simulink model "Trajectory_Tracking_Control_Structure3_Modifying"  (R2017b)
settings: Solver=VariableStepAuto  StartTime=0  StopTime=times(end)  RelTol=1e-6
values from neighbouring files (symbols this model uses):
  a_piecewise = zeros(max(DOF_a_piecewise),length(DOF_a_piecewise))    [Trajectory_Generator_Minimum_Snap.m]
  b_piecewise = zeros(max(DOF_b_piecewise),length(DOF_b_piecewise))    [Trajectory_Generator_Minimum_Snap.m]
  c_piecewise = zeros(max(DOF_c_piecewise),length(DOF_c_piecewise))    [Trajectory_Generator_Minimum_Snap.m]
  d_piecewise = zeros(max(DOF_d_piecewise),length(DOF_d_piecewise))    [Trajectory_Generator_Minimum_Snap.m]
settings Model: Creator=chenjiasheng  LastModifiedBy=chenjiasheng

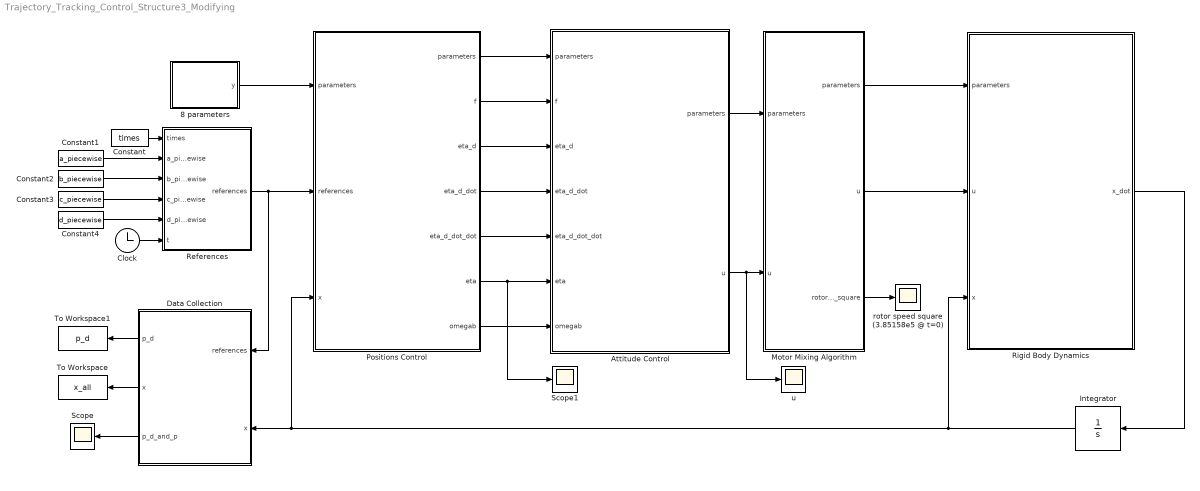
== system Trajectory_Tracking_Control_Structure3_Modifying ==
  8 parameters : MATLAB Function  TreatAsAtomicUnit=on
  Attitude Control : MATLAB Function  TreatAsAtomicUnit=on
  Clock : Clock
  Constant : Constant  Value=times
  Constant1 : Constant  Value=a_piecewise
  Constant2 : Constant  Value=b_piecewise
  Constant3 : Constant  Value=c_piecewise
  Constant4 : Constant  Value=d_piecewise
  Data Collection : MATLAB Function  TreatAsAtomicUnit=on
  Integrator : Integrator  InitialCondition=[0 0 0, 0 0 0, 0 0 0, 0 0 0]  ContinuousStateAttributes='x'
  Motor Mixing Algorithm : MATLAB Function  TreatAsAtomicUnit=on
  Positions Control : MATLAB Function  TreatAsAtomicUnit=on
  References : MATLAB Function  TreatAsAtomicUnit=on
  Rigid Body Dynamics : MATLAB Function  TreatAsAtomicUnit=on
  Scope : Scope
  Scope1 : Scope
  To Workspace : ToWorkspace  VariableName=x_all  SampleTime=0.01
  To Workspace1 : ToWorkspace  VariableName=p_d  SampleTime=0.01
  rotor speed square (3.85158e5 @ t=0) : Scope
  u : Scope
  wires:
  8 parameters/1(y) -> Positions Control/1("parameters ")
  References/1(references) -> Positions Control/2(references), Data Collection/1(references)
  Positions Control/1(parameters) -> Attitude Control/1("parameters ")
  Positions Control/2(f) -> Attitude Control/2(f)
  Positions Control/3(eta_d) -> Attitude Control/3(eta_d)
  Positions Control/4(eta_d_dot) -> Attitude Control/4(eta_d_dot)
  Rigid Body Dynamics/1(x_dot) -> Integrator/1
  Integrator/1 -> Rigid Body Dynamics/3(x), Positions Control/3(x), Data Collection/2("x ")
  Attitude Control/1(parameters) -> Motor Mixing Algorithm/1("parameters ")
  Attitude Control/2(u) -> u/1, Motor Mixing Algorithm/2("u ")
  Clock/1 -> References/6(t)
  Motor Mixing Algorithm/1(parameters) -> Rigid Body Dynamics/1(parameters)
  Motor Mixing Algorithm/2(u) -> Rigid Body Dynamics/2(u)
  Motor Mixing Algorithm/3(rotor_speed_square) -> rotor speed square (3.85158e5 @ t=0)/1
  Positions Control/5(eta_d_dot_dot) -> Attitude Control/5(eta_d_dot_dot)
  Positions Control/6(eta) -> Scope1/1, Attitude Control/6(eta)
  Positions Control/7(omegab) -> Attitude Control/7(omegab)
  Constant/1 -> References/1(times)
  Constant1/1 -> References/2(a_piecewise)
  Constant2/1 -> References/3(b_piecewise)
  Constant3/1 -> References/4(c_piecewise)
  Constant4/1 -> References/5(d_piecewise)
  Data Collection/1(p_d) -> To Workspace1/1
  Data Collection/3(p_d_and_p) -> Scope/1
  Data Collection/2(x) -> To Workspace/1

== matlab function Trajectory_Tracking_Control_Structure3_Modifying/Positions Control ==
  data: parameters input size=8; parameters output size=8; references input size=18; x input size=12; f output size=1; eta_d output size=3; eta_d_dot output size=3; eta_d_dot_dot output size=3; eta output size=3; omegab output size=3
 function [parameters,f,eta_d,eta_d_dot,eta_d_dot_dot,eta,omegab] =fcn(parameters,references,x)
%% kp,kd for the positions controller
Kp=diag([0 0 0]); % Kp=diag([kpx kpy kpz]) [20 30 20]
Kd=diag([0 0 0]);    % Kd=diag([kdx kdy kdz])[6 15 6]
%% allocate inputs
m=parameters(1);
g=parameters(2);
p_d=references(1:3);   % reference's positions
v_d=references(4:6);   % reference's velocities
a_d=references(7:9);   % reference's accelerations
a_d_dot=references(10:12);    % reference's jerk
a_d_dot_dot=references(13:15);% reference's snap
psi_d=references(16);         % reference's yaw angle 
psi_d_dot=references(17);     % reference's change rate of the yaw angle
psi_d_dot_dot=references(18); % reference's change rate of change rate of the yaw angle
p=x(1:3) ;     % positions 
v=x(4:6) ;     % velocities
eta=x(7:9);    % euler angle
omegab=x(10:12); 
phi=eta(1);
theta=eta(2);
psi=eta(3);
Rbn=[cos(theta)*cos(psi) sin(phi)*sin(theta)*cos(psi)-cos(phi)*sin(psi) cos(phi)*sin(theta)*cos(psi)+sin(phi)*sin(psi);
     cos(theta)*sin(psi) sin(phi)*sin(theta)*sin(psi)+cos(phi)*cos(psi) cos(phi)*sin(theta)*sin(psi)-sin(phi)*cos(psi);
     -sin(theta)         sin(phi)*cos(theta)                            cos(phi)*cos(theta)                           ];
zb=Rbn(:,3);
%% acceleration, jerk, snap control
a_c=Kp*(p_d-p)+Kd*(v_d-v)+a_d;  % acceleration of control
f=m*sqrt(a_c(1)^2+a_c(2)^2+(g+a_c(3))^2);
a=1/m*Rbn*[0 0 f]'-[0 0 g]';
a_c_dot=Kp*(v_d-v)+Kd*(a_d-a)+a_d_dot ;   % acceleration of control dot
a_dot=m/f*[a_c(1),a_c(2),a_c(3)+g]*a_c_dot*zb+f/m*cross((Rbn*omegab),zb);
a_c_dot_dot=Kp*(a_d-a)+Kd*(a_d_dot-a_dot)+a_d_dot_dot; % acceleration of control dot dot
%% define some variables to make our life easier
A=a_c(1)*sin(psi_d)-a_c(2)*cos(psi_d); 
C=a_c(1)*cos(psi_d)+a_c(2)*sin(psi_d);
D=g+a_c(3);
B=sqrt(C^2+D^2);
A_dot=sin(psi_d)*a_c_dot(1)-cos(psi_d)*a_c_dot(2)+C*psi_d_dot;                                   
C_dot=cos(psi_d)*a_c_dot(1)+sin(psi_d)*a_c_dot(2)-A*psi_d_dot;                                  
D_dot=a_c_dot(3);                                                                                
B_dot=(C*C_dot+D*D_dot)/B;  
fbmsd=2*a_c(1)*a_c_dot(1)+2*a_c(2)*a_c_dot(2)+2*(g+a_c(3))*a_c_dot(3);   % f by m square dot
%% phi_d, theta_d 
phi_d=asin(A*m/f) ;
theta_d=sign(C)*acos(D/B);
%% phi_d_dot,theta_d_dot
phi_d_dot=(sin(psi_d)*(f/m)^2-A*a_c(1))/((f/m)^2*B)*a_c_dot(1) + (-cos(psi_d)*(f/m)^2-A*a_c(2))/((f/m)^2*B)*a_c_dot(2) + (-A*D)/((f/m)^2*B)*a_c_dot(3) + C/B*psi_d_dot ;
theta_d_dot=(cos(psi_d)*D*a_c_dot(1)+sin(psi_d)*D*a_c_dot(2)-C*a_c_dot(3)-A*D*psi_d_dot)/B^2   ; 
%% phi_d_dot_dot, theta_d_dot_dot
monster11=(cos(psi_d)*psi_d_dot*(f/m)^2+sin(psi_d)*fbmsd-(A_dot*a_c(1)+A*a_c_dot(1)))*a_c_dot(1)+(sin(psi_d)*(f/m)^2-A*a_c(1))*a_c_dot_dot(1);
monster12=(-sin(psi_d)*psi_d_dot*(f/m)^2+cos(psi_d)*fbmsd+A_dot*a_c(2)+A*a_c_dot(2))*a_c_dot(2)+(cos(psi_d)*(f/m)^2+A*a_c(2))*a_c_dot_dot(2);
monster13=(A_dot*D+A*D_dot)*a_c_dot(3)+A*D*a_c_dot_dot(3);
monster1=monster11-monster12-monster13;
phi_d_dot_dot=(monster1-(B*phi_d_dot-C*psi_d_dot)*fbmsd)/((f/m)^2*B) + (C_dot*psi_d_dot+C*psi_d_dot_dot-B_dot*phi_d_dot)/B;
monster21=(-sin(psi_d)*psi_d_dot*D+cos(psi_d)*D_dot)*a_c_dot(1)+cos(psi_d)*D*a_c_dot_dot(1);
monster22=(cos(psi_d)*psi_d_dot*D+sin(psi_d)*D_dot)*a_c_dot(2)+sin(psi_d)*D*a_c_dot_dot(2);
monster23= C_dot*a_c_dot(3)+C*a_c_dot_dot(3);
monster24=(A_dot*D+A*D_dot)*psi_d_dot+A*D*psi_d_dot_dot;
monster2= monster21+monster22-monster23-monster24;
theta_d_dot_dot=monster2/B^2-2*theta_d_dot*B_dot/B;
%% output eta_d, eta_d_dot, eta_d_dot_dot                        
 % output 1-8: eight parameters  (given above)
 % output 9: f (given above)
eta_d=[phi_d;theta_d;psi_d]   ;                 % output 10-12
eta_d_dot=[phi_d_dot;theta_d_dot;psi_d_dot] ;       % output 13-15 
eta_d_dot_dot=[phi_d_dot_dot;theta_d_dot_dot;psi_d_dot_dot];% output 16-18
 % output 19-21: eta (given above)
 % output 22-24: omegab (given above)

== matlab function Trajectory_Tracking_Control_Structure3_Modifying/8 parameters ==
  data: y output size=8
function y=fcn
%% specify parameters
m=0.468;
g=9.81;
Ix=4.856*10^(-3);
Iy=4.856*10^(-3);
Iz=8.801*10^(-3);
l=0.225;
k=2.980*10^-6;
c=1.140*10^-7;
%% output
y=[m;g;Ix;Iy;Iz;l;k;c]; % output # 1-8
    
end

== matlab function Trajectory_Tracking_Control_Structure3_Modifying/Attitude Control ==
  data: parameters input size=8; parameters output size=8; f input size=1; eta_d input size=3; eta_d_dot input size=3; eta_d_dot_dot input size=3; eta input size=3; omegab input size=3; u output size=4
function [parameters,u]=fcn(parameters,f,eta_d,eta_d_dot,eta_d_dot_dot,eta,omegab)
%% kp, kd for the attitude control
KP=diag([150 150 150]); % kp_phi, kp_theta, kp_psi
KD=diag([22 22 22]); % kd_phi, kd_theta, kd_psi
%% allocate inputs
M=diag([parameters(3), parameters(4), parameters(5)]);
phi=eta(1);
theta=eta(2);
psi=eta(3);
eta_dot=[1 sin(phi)*tan(theta) cos(phi)*tan(theta);
         0 cos(phi)            -sin(phi);
         0 sin(phi)/cos(theta) cos(phi)/cos(theta)]*omegab;
phi_dot=eta_dot(1);
theta_dot=eta_dot(2);
psi_dot=eta_dot(3);
%% get taub
eta_c_dot_dot=KP*(eta_d-eta)+KD*(eta_d_dot-eta_dot)+eta_d_dot_dot;
phi_c_dot_dot=eta_c_dot_dot(1);
theta_c_dot_dot=eta_c_dot_dot(2);
psi_c_dot_dot=eta_c_dot_dot(3);
p_c_dot=phi_c_dot_dot-psi_c_dot_dot*sin(theta)-theta_dot*psi_dot*cos(theta);
q_c_dot=theta_c_dot_dot*cos(phi)+psi_c_dot_dot*sin(phi)*cos(theta)-phi_dot*theta_dot*sin(phi)+phi_dot*psi_dot*cos(phi)*cos(theta)-theta_dot*psi_dot*sin(phi)*sin(theta);
r_c_dot=-theta_c_dot_dot*sin(phi)+psi_c_dot_dot*cos(phi)*cos(theta)-phi_dot*theta_dot*cos(phi)-phi_dot*psi_dot*sin(phi)*cos(theta)-theta_dot*psi_dot*cos(phi)*sin(theta);
omegab_c_dot=[p_c_dot q_c_dot r_c_dot]' ;
taub=M*omegab_c_dot+cross(omegab,M*omegab); 
%% u
u=[f;taub]; % here I should use " f_c, taub_c " maybe in the future if I do rotor dynamics

end

== matlab function Trajectory_Tracking_Control_Structure3_Modifying/References ==
  data: times input; a_piecewise input; b_piecewise input; c_piecewise input; d_piecewise input; t input size=1; references output size=18
function references = fcn(times,a_piecewise,b_piecewise,c_piecewise,d_piecewise,t)
% to speed up computation, I can move the code below into "Trajectory_Generator" as many as possbible, but it's OK temporarily.
%% In short, determine where we are
if t==times(end)
which_piece=length(times)-1;
else
which_piece=length(find(times<=t));
end
a_piece=a_piecewise(:,which_piece);
b_piece=b_piecewise(:,which_piece);
c_piece=c_piecewise(:,which_piece);
d_piece=d_piecewise(:,which_piece);
%% flip,take derivative for the final computation
a_piece_flip=flip(a_piece);
a_piece_flip_dot=polyder(a_piece_flip);
a_piece_flip_dot2=polyder(a_piece_flip_dot);
a_piece_flip_dot3=polyder(a_piece_flip_dot2);
a_piece_flip_dot4=polyder(a_piece_flip_dot3);
%--------------------------------------------------------------------------
b_piece_flip=flip(b_piece);
b_piece_flip_dot=polyder(b_piece_flip);
b_piece_flip_dot2=polyder(b_piece_flip_dot);
b_piece_flip_dot3=polyder(b_piece_flip_dot2);
b_piece_flip_dot4=polyder(b_piece_flip_dot3);
%--------------------------------------------------------------------------
c_piece_flip=flip(c_piece);
c_piece_flip_dot=polyder(c_piece_flip);
c_piece_flip_dot2=polyder(c_piece_flip_dot);
c_piece_flip_dot3=polyder(c_piece_flip_dot2);
c_piece_flip_dot4=polyder(c_piece_flip_dot3);
%--------------------------------------------------------------------------
d_piece_flip=flip(d_piece);
d_piece_flip_dot=polyder(d_piece_flip);
d_piece_flip_dot2=polyder(d_piece_flip_dot);
%% compute references
p_d=[polyval(a_piece_flip,t),polyval(b_piece_flip,t),polyval(c_piece_flip,t)]'    ;             % reference's positions
v_d=[polyval(a_piece_flip_dot,t),polyval(b_piece_flip_dot,t),polyval(c_piece_flip_dot,t)]'    ;        % reference's velocities
a_d=[polyval(a_piece_flip_dot2,t),polyval(b_piece_flip_dot2,t),polyval(c_piece_flip_dot2,t)]'   ;        % reference's accelerations
a_d_dot=[polyval(a_piece_flip_dot3,t),polyval(b_piece_flip_dot3,t),polyval(c_piece_flip_dot3,t)]';      % reference's jerk
a_d_dot_dot=[polyval(a_piece_flip_dot4,t),polyval(b_piece_flip_dot4,t),polyval(c_piece_flip_dot4,t)]';   % reference's snap
psi_d= polyval(d_piece_flip,t) ;            % reference's yaw angle
psi_d_dot= polyval(d_piece_flip_dot,t) ;            % reference's change rate of yaw angle
psi_d_dot_dot= polyval(d_piece_flip_dot2,t)    ;            % reference's change rate of change rate of yaw angle

references=[ p_d;           %  1-3
             v_d;           %  4-6
             a_d;           %  7-9
             a_d_dot;       %  10-12
             a_d_dot_dot;   %  13-15
             psi_d;         %  16
             psi_d_dot;     %  17
             psi_d_dot_dot];%  18  
end

== matlab function Trajectory_Tracking_Control_Structure3_Modifying/Motor Mixing Algorithm ==
  data: parameters output; u output; parameters input size=8; u input size=4; rotor_speed_square output size=4
function [parameters,u,rotor_speed_square]=fcn(parameters,u)
l=parameters(6) ; 
k=parameters(7) ;
c=parameters(8) ;
rotor_speed_square=[1 0 -1  1;
                    1 1  0 -1;
                    1 0  1  1;
                    1 -1 0 -1]* [1/(4*k) 0         0         0;
                                0        1/(2*l*k) 0         0;
                                0        0         1/(2*l*k) 0;
                                0        0         0         1/(4*c)]*u ;
end
%% Motor dynamics
% rotor_speed=in(9:12)
% rotor_speed_square=rotor_speed.^2
%f_taux_tauy_tauz=[k 0   0   0;
%                  0 k*l 0   0;
%                  0 0   k*l 0;
%                  0 0   0   c]*[1  1 1  1;
%                                0  1 0 -1;
%                               -1  0 1  0;
%                                1 -1 1 -1]*rotor_speed_square

== matlab function Trajectory_Tracking_Control_Structure3_Modifying/Rigid Body Dynamics ==
  data: parameters input size=8; x_dot output size=12; u input size=4; x input size=12
function x_dot=fcn(parameters,u,x)
%% allocate inputs
m=parameters(1);
g=parameters(2);
M=diag([parameters(3) parameters(4) parameters(5)]);
f=u(1);
taub=u(2:4);
pn=x(1:3);
vn=x(4:6);
eta=x(7:9);
omegab=x(10:12);
%% define matrix Rbn , Lbn and Omega
phi=eta(1);
theta=eta(2);
psi=eta(3);
Rbn=[cos(theta)*cos(psi) sin(phi)*sin(theta)*cos(psi)-cos(phi)*sin(psi) cos(phi)*sin(theta)*cos(psi)+sin(phi)*sin(psi);
     cos(theta)*sin(psi) sin(phi)*sin(theta)*sin(psi)+cos(phi)*cos(psi) cos(phi)*sin(theta)*sin(psi)-sin(phi)*cos(psi);
     -sin(theta)         sin(phi)*cos(theta)                            cos(phi)*cos(theta)                           ];
Lbn=[1 sin(phi)*tan(theta) cos(phi)*tan(theta);
     0 cos(phi)            -sin(phi);
     0 sin(phi)/cos(theta) cos(phi)/cos(theta)];

%% nonlinear model: shown on the handout
pn_dot=vn;
vn_dot=1/m*Rbn*[0 0 f]'-[0 0 g]'; % -1/m*[Ax 0 0;0 Ay 0;0 0 Az]*pn_dot;    % pay attention to whether I need Ax, Ay, Az
eta_dot=Lbn*omegab;
omegab_dot=M\(taub-cross(omegab,M*omegab));
%% output x_dot
x_dot=[pn_dot;
       vn_dot;
       eta_dot;
       omegab_dot];
end

== matlab function Trajectory_Tracking_Control_Structure3_Modifying/Data Collection ==
  data: references input; p_d output; x output; x input; p_d_and_p output
function [p_d,x,p_d_and_p] = Data_Collection(references,x)
% This block are used for data collection. Modify inputs and outputs anytime as needed.
p_d=references(1:3);
p_d_and_p=[p_d;x(1:3)];
end
